simulink model "myClassification2In2Mid2Out"  (R2024a)
settings: Solver=FixedStepDiscrete  StartTime=0.0  StopTime=1  FixedStep=1  MaxStep=1  RelTol=1e-3
InitFcn:
  | close all;
  | clear all;
  | % 入力格子（行列）作成
  | [x1, x2] = meshgrid(-1.2:0.1:1.2, -1.2:0.1:1.2);
  | y = zeros(10, 10);
StopFcn:
  | y = out.y.Data;
  | figure;
  | % y1 < y2の時赤プロット
  | scatter(x1(y == true), x2(y == true), ...
  |     'filled', 'r');
  | hold on
  | % y2 <= y1の時青プロット
  | scatter(x1(y == false), x2(y == false), ...
  |     'filled', 'b');
  | grid on
undefined symbols (not defined in the file or in its folder): x1, x2
libraries: neural x2
settings Model: Creator=mashi  LastModifiedBy=mashi

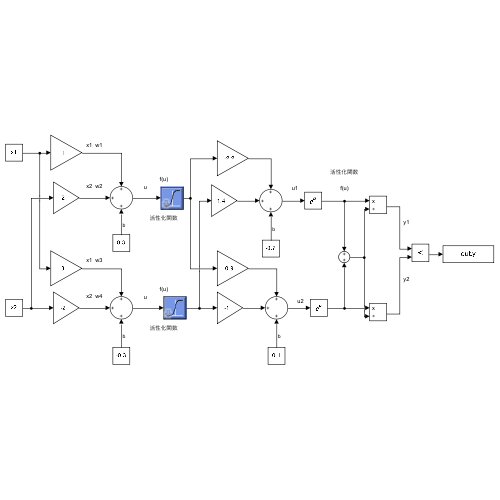
[thumbnail: Simulink's stored preview of the top-level diagram]
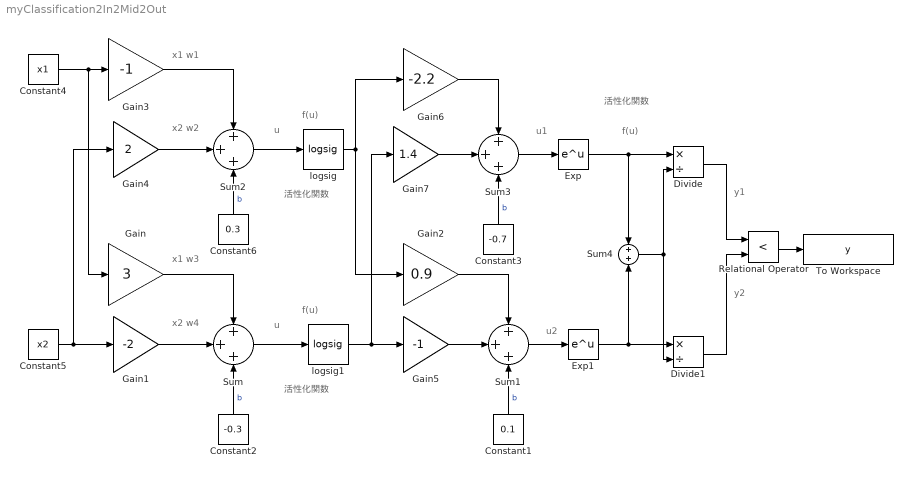
== system myClassification2In2Mid2Out ==
  note: 活性化関数
  note: u
  note: f(u)
  note: x2 w4
  note: x1 w3
  note: 活性化関数
  note: u
  note: f(u)
  note: x2 w2
  note: x1 w1
  note: u2
  note: f(u)
  note: 活性化関数
  note: u1
  note: y1
  note: y2
  Constant1 : Constant  Value=0.1
  Constant2 : Constant  Value=-0.3
  Constant3 : Constant  Value=-0.7
  Constant4 : Constant  Value=x1
  Constant5 : Constant  Value=x2
  Constant6 : Constant  Value=0.3
  Divide : Product  Inputs=*/
  Divide1 : Product  Inputs=*/
  Exp : Math
  Exp1 : Math
  Gain : Gain  Gain=3
  Gain1 : Gain  Gain=-2
  Gain2 : Gain  Gain=0.9
  Gain3 : Gain  Gain=-1
  Gain4 : Gain  Gain=2
  Gain5 : Gain  Gain=-1
  Gain6 : Gain  Gain=-2.2
  Gain7 : Gain  Gain=1.4
  Relational Operator : RelationalOperator  Operator=<  OutDataTypeStr=boolean  RndMeth=Simplest  InputSameDT=off
  Sum{,1..3} (4 alike) : Sum  Inputs=+++
  Sum4 : Sum
  To Workspace : ToWorkspace  VariableName=y  SaveFormat=Timeseries  SampleTime=-1
  logsig : neural/Transfer Functions/logsig
  logsig1 : neural/Transfer Functions/logsig
  wires:
  Gain/1 -> Sum/1
  Gain1/1 -> Sum/2
  Constant2/1 -> Sum/3  "b"
  Constant6/1 -> Sum2/3  "b"
  Gain4/1 -> Sum2/2
  Gain3/1 -> Sum2/1
  Constant4/1 -> Gain/1, Gain3/1
  Constant5/1 -> Gain4/1, Gain1/1
  Sum2/1 -> logsig/1
  Sum/1 -> logsig1/1
  Sum1/1 -> Exp1/1
  Sum3/1 -> Exp/1
  Gain6/1 -> Sum3/1
  Gain7/1 -> Sum3/2
  Constant3/1 -> Sum3/3  "b"
  Constant1/1 -> Sum1/3  "b"
  Gain5/1 -> Sum1/2
  Gain2/1 -> Sum1/1
  logsig1/1 -> Gain7/1, Gain5/1
  logsig/1 -> Gain6/1, Gain2/1
  Exp/1 -> Sum4/1, Divide/1
  Exp1/1 -> Sum4/2, Divide1/1
  Sum4/1 -> Divide1/2, Divide/2
  Divide/1 -> Relational Operator/1
  Divide1/1 -> Relational Operator/2
  Relational Operator/1 -> To Workspace/1
